simulink model "regulatorPID"  (R2018a)
settings: Solver=VariableStepAuto  StartTime=0.0  StopTime=3  RelTol=1e-3
settings Model: Creator=ilier  LastModifiedBy=ilier

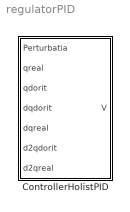
== system regulatorPID ==
  ControllerHolistPID : Subsystem

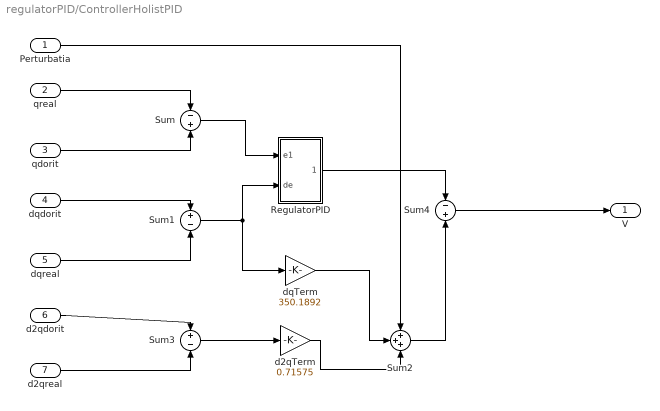
== system regulatorPID/ControllerHolistPID ==
  Perturbatia : Inport
  qreal : Inport  Port=2
  qdorit : Inport  Port=3
  dqdorit : Inport  Port=4
  dqreal : Inport  Port=5
  "d2qdorit " : Inport  Port=6
  d2qreal : Inport  Port=7
  RegulatorPID : Subsystem
  Sum : Sum  Inputs=-+
  Sum1 : Sum  Inputs=+-
  Sum2 : Sum  Inputs=+++
  Sum3 : Sum  Inputs=+-
  Sum4 : Sum  Inputs=-+
  "d2qTerm " : Gain  Gain=0.71575
  dqTerm : Gain  Gain=350.1892
  V : Outport
  wires:
  qreal/1 -> Sum/1
  dqreal/1 -> Sum1/2
  qdorit/1 -> Sum/2
  "d2qdorit "/1 -> Sum3/1
  dqTerm/1 -> Sum2/2
  Sum3/1 -> "d2qTerm "/1
  Sum/1 -> RegulatorPID/1(e1)
  Sum4/1 -> V/1
  Perturbatia/1 -> Sum2/1
  dqdorit/1 -> Sum1/1
  "d2qTerm "/1 -> Sum2/3
  Sum1/1 -> dqTerm/1, RegulatorPID/2(de)
  RegulatorPID/1(u*1) -> Sum4/1
  Sum2/1 -> Sum4/2
  d2qreal/1 -> Sum3/2

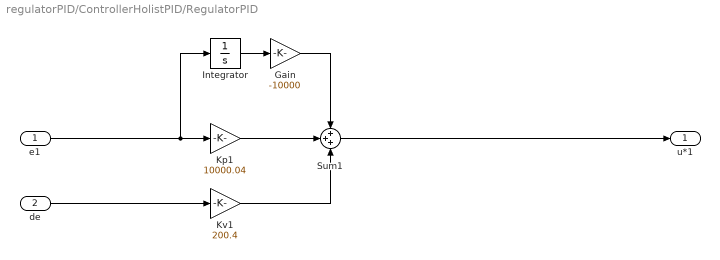
== system regulatorPID/ControllerHolistPID/RegulatorPID ==
  e1 : Inport
  de : Inport  Port=2
  Gain : Gain  Gain=-10000
  Integrator : Integrator
  Kp1 : Gain  Gain=10000.04
  Kv1 : Gain  Gain=200.4
  Sum1 : Sum  Inputs=+++
  u*1 : Outport
  wires:
  de/1 -> Kv1/1
  e1/1 -> Integrator/1, Kp1/1
  Kv1/1 -> Sum1/3
  Kp1/1 -> Sum1/2
  Sum1/1 -> u*1/1
  Gain/1 -> Sum1/1
  Integrator/1 -> Gain/1
